simulink model "fourier"  (Simulink 5.0)
settings: Solver=ode45  StartTime=0.0  StopTime=10.0  RelTol=1e-3
values from neighbouring files (symbols this model uses):
  x = x + s    [broyden.m]    (also in broyden1.m = x+s; dominio.m = A1*sin(2*pi*fc*t)+A1*cos(2*pi*fc*t); grafica.m = xo; graficaquiz.m = [-20:1:20])
undefined symbols (not defined in the file or in its folder): get
libraries: dspsnks4 x1
settings Model: LastModifiedBy=Invitado

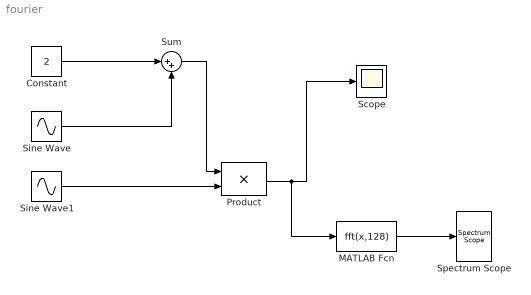
== system fourier ==
  Constant : Constant  Value=2
  MATLAB Fcn : MATLABFcn  MATLABFcn=fft(x,128)
  Product : Product  SaturateOnIntegerOverflow=on
  Scope : Scope
  Sine Wave : Sin  Amplitude=2  SampleTime=0.01
  Sine Wave1 : Sin  Amplitude=2  Frequency=20  SampleTime=0.01
  Spectrum Scope : dspsnks4/Spectrum Scope  ScopeProperties=on  Domain=Frequency  HorizSpan=1  UseBuffer=off  BufferSize=128  Overlap=64  inpFftLenInherit=off  FFTlength=128  numAvg=2  DisplayProperties=off  AxisGrid=on  Memory=off  FrameNumber=on  AxisLegend=off  AxisZoom=off  OpenScopeAtSimStart=on  OpenScopeImmediately=off  FigPos=get(0,'defaultfigureposition')  AxisProperties=off  XUnits=Hertz  XRange=[0...Fs/2]  InheritXIncr=on  XIncr=1.0  XLabel=Samples  YUnits=dB  YLabel=Magnitude, dB  LineProperties=off
      settings: YMin=-164.362377632534  YMax=32.9892476196018
  Sum : Sum  Inputs=|++  SaturateOnIntegerOverflow=on
  wires:
  Constant/1 -> Sum/1
  Sine Wave/1 -> Sum/2
  Sum/1 -> Product/1
  Sine Wave1/1 -> Product/2
  Product/1 -> Scope/1, MATLAB Fcn/1
  MATLAB Fcn/1 -> Spectrum Scope/1
